simulink model "case2_16Ae10005"  (R2017b)
settings: Solver=ode4  StartTime=0.0  StopTime=10.0  FixedStep=0.0001  RelTol=1e-3
libraries: simulink x1
settings Model: Creator=ayushi  LastModifiedBy=ayushi

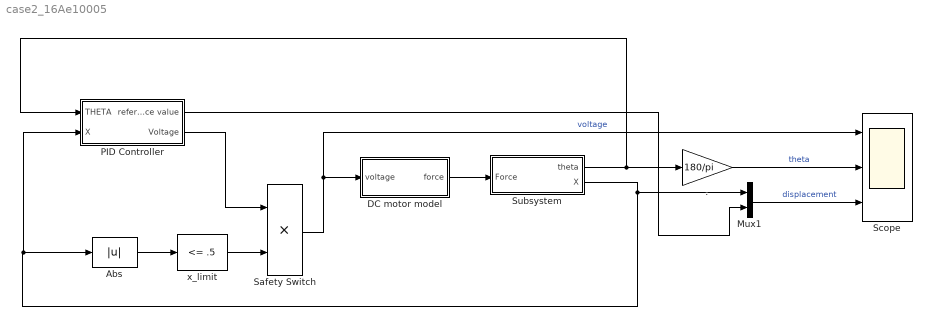
== system case2_16Ae10005 ==
  ". " : Gain  Gain=180/pi
  Abs : Abs
  DC motor model : Subsystem
  Mux1 : Mux  Inputs=2
  "PID Controller " : Subsystem
  Safety Switch : Product
  Scope : Scope  NumInputPorts=3
  Subsystem : Subsystem
  x_limit : simulink/Logic and Bit Operations/Compare To Constant  relop=<=  const=.5  OutDataTypeStr=boolean
  wires:
  Subsystem/1("theta ") -> "PID Controller "/1(THETA), ". "/1
  Abs/1 -> x_limit/1
  "PID Controller "/2(Voltage) -> Safety Switch/1
  DC motor model/1(force) -> Subsystem/1(Force)
  ". "/1 -> Scope/2  "theta"
  x_limit/1 -> Safety Switch/2
  Safety Switch/1 -> Scope/1, DC motor model/1(voltage)  "voltage"
  Subsystem/2("X ") -> Abs/1, "PID Controller "/2(X), Mux1/1
  Mux1/1 -> Scope/3  "displacement"
  "PID Controller "/1(reference value) -> Mux1/2

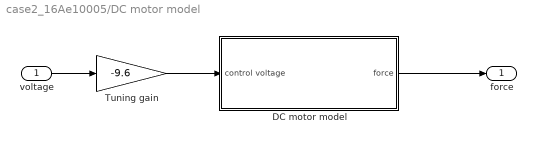
== system case2_16Ae10005/DC motor model ==
  voltage : Inport
  DC motor model : Subsystem  mask{J=0.0000140, Kt=0.05, Kb=0.05, d=0.000001, R=2.5, L=0.0025}
      mask prompts: J "Moment of inertia"; Kt "Torque constant"; Kb "Electromotive force constant"; d "Linear approximation of viscous friction"; R "Electrical circuit resistance"; L "Electrical circuit inductance"
      mask Display: disp('DC motor')
  Tuning gain : Gain  Gain=-9.6
  force : Outport
  wires:
  Tuning gain/1 -> DC motor model/1(control voltage)
  voltage/1 -> Tuning gain/1
  DC motor model/1(force) -> force/1

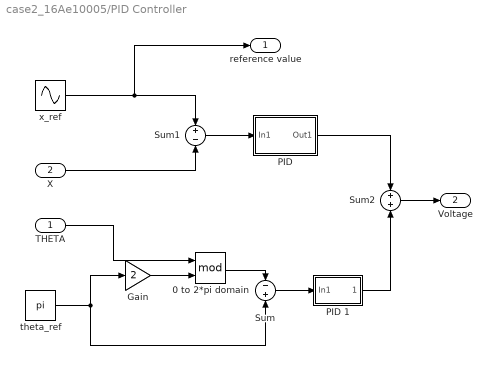
== system case2_16Ae10005/PID Controller  ==
  THETA : Inport
  X : Inport  Port=2
  0 to 2*pi domain : Math  Operator=mod  SaturateOnIntegerOverflow=on
  Gain : Gain  Gain=2
  "PID " : Subsystem
  PID 1 : Subsystem
  Sum : Sum  Inputs=-+
  Sum1 : Sum  Inputs=+-
  Sum2 : Sum
  theta_ref : Constant  Value=pi
  x_ref : Sin  Amplitude=.25  Frequency=pi/4  SampleTime=0
  reference value : Outport
  Voltage : Outport  Port=2
  wires:
  theta_ref/1 -> Gain/1, Sum/2
  THETA/1 -> 0 to 2*pi domain/1
  0 to 2*pi domain/1 -> Sum/1
  "PID "/1(Out1) -> Sum2/1
  Sum2/1 -> Voltage/1
  X/1 -> Sum1/2
  x_ref/1 -> reference value/1, Sum1/1
  Sum1/1 -> "PID "/1(In1)
  Sum/1 -> PID 1/1(In1)
  PID 1/1(Out1) -> Sum2/2
  Gain/1 -> 0 to 2*pi domain/2

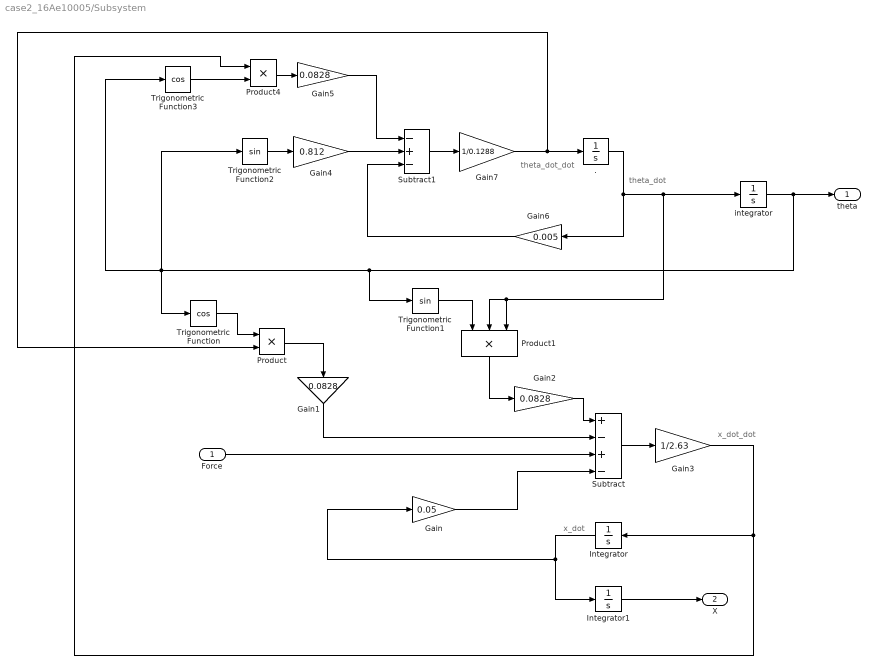
== system case2_16Ae10005/Subsystem ==
  note: theta_dot
  note: theta_dot_dot
  note: x_dot
  note: x_dot_dot
  Force : Inport
  ". " : Integrator
  Gain : Gain  Gain=0.05
  Gain1 : Gain  Gain=0.0828
  Gain2 : Gain  Gain=0.0828
  Gain3 : Gain  Gain=1/2.63
  Gain4 : Gain  Gain=0.812
  Gain5 : Gain  Gain=0.0828
  Gain6 : Gain  Gain=0.005
  Gain7 : Gain  Gain=1/0.1288
  Integrator : Integrator
  Integrator1 : Integrator
  Product : Product
  Product1 : Product  Inputs=3
  Product4 : Product
  Subtract : Sum  Inputs=+-+-
  Subtract1 : Sum  Inputs=-+-
  Trigonometric Function : Trigonometry  Operator=cos
  Trigonometric Function1 : Trigonometry
  Trigonometric Function2 : Trigonometry
  Trigonometric Function3 : Trigonometry  Operator=cos
  integrator : Integrator
  "theta " : Outport
  "X " : Outport  Port=2
  wires:
  Trigonometric Function2/1 -> Gain4/1
  Integrator1/1 -> "X "/1
  integrator/1 -> "theta "/1, Trigonometric Function1/1, Trigonometric Function3/1, Trigonometric Function/1, Trigonometric Function2/1
  Gain/1 -> Subtract/4
  Integrator/1 -> Gain/1, Integrator1/1
  Gain3/1 -> Product4/1, Integrator/1
  Gain7/1 -> Product/2, ". "/1
  Product/1 -> Gain1/1
  Gain4/1 -> Subtract1/2
  Force/1 -> Subtract/3
  Product4/1 -> Gain5/1
  Trigonometric Function/1 -> Product/1
  Trigonometric Function1/1 -> Product1/1
  Trigonometric Function3/1 -> Product4/2
  Gain6/1 -> Subtract1/3
  ". "/1 -> Gain6/1, Product1/3, Product1/2, integrator/1
  Product1/1 -> Gain2/1
  Gain2/1 -> Subtract/1
  Gain1/1 -> Subtract/2
  Gain5/1 -> Subtract1/1
  Subtract/1 -> Gain3/1
  Subtract1/1 -> Gain7/1

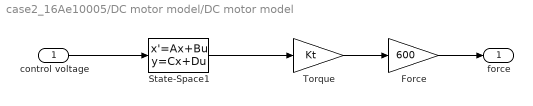
== system case2_16Ae10005/DC motor model/DC motor model ==
  control voltage : Inport
  Force : Gain  Gain=600
  State-Space1 : StateSpace  A=[-d/J Kt/J;-Kb/L -R/L]  B=[0; 1/L]  C=[0 1]  D=0  InitialCondition=0
  Torque : Gain  Gain=Kt
  force : Outport
  wires:
  control voltage/1 -> State-Space1/1
  State-Space1/1 -> Torque/1
  Torque/1 -> Force/1
  Force/1 -> force/1

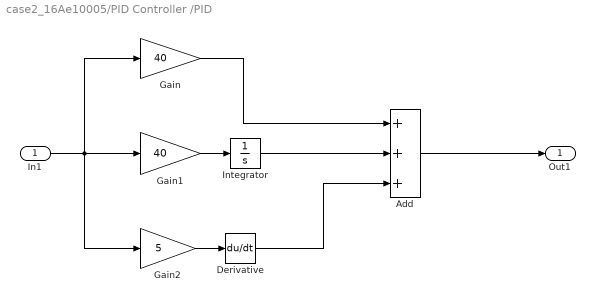
== system case2_16Ae10005/PID Controller /PID  ==
  In1 : Inport
  Add : Sum  Inputs=+++
  Derivative : Derivative
  Gain : Gain  Gain=40
  Gain1 : Gain  Gain=40
  Gain2 : Gain  Gain=5
  Integrator : Integrator
  Out1 : Outport
  wires:
  Gain/1 -> Add/1
  Gain2/1 -> Derivative/1
  Derivative/1 -> Add/3
  Integrator/1 -> Add/2
  Add/1 -> Out1/1
  In1/1 -> Gain2/1, Gain1/1, Gain/1
  Gain1/1 -> Integrator/1

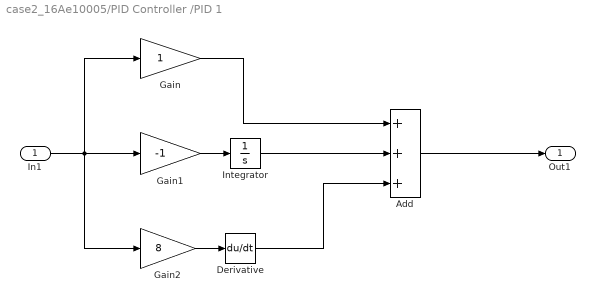
== system case2_16Ae10005/PID Controller /PID 1 ==
  In1 : Inport
  Add : Sum  Inputs=+++
  Derivative : Derivative
  Gain : Gain
  Gain1 : Gain  Gain=-1
  Gain2 : Gain  Gain=8
  Integrator : Integrator
  Out1 : Outport
  wires:
  Gain/1 -> Add/1
  Gain2/1 -> Derivative/1
  Derivative/1 -> Add/3
  Integrator/1 -> Add/2
  Add/1 -> Out1/1
  In1/1 -> Gain2/1, Gain1/1, Gain/1
  Gain1/1 -> Integrator/1
